simulink model "linearizzazione_pendolo_inv"  (R2020b)
settings: Solver=VariableStepAuto  StartTime=0.0  StopTime=20.0  RelTol=1e-3
values from neighbouring files (symbols this model uses):
  A = [0 1; -k/(m*L*L)+g/L*cos(x_bar(1)) -a/(m*L*L)]    [pendolo_inverso.m]
  B = [0 ; 0]    [pendolo_inverso.m]
  C = [1 0]    [pendolo_inverso.m]
  D = 0    [pendolo_inverso.m]
  du = u-u_bar    (= 0)    [pendolo_inverso.m]
  dx0 = x0-x_bar    [pendolo_inverso.m]
  x_bar = [0.713; 0]    [pendolo_inverso.m]
settings Model: Creator=Lenovo  LastModifiedBy=Lenovo

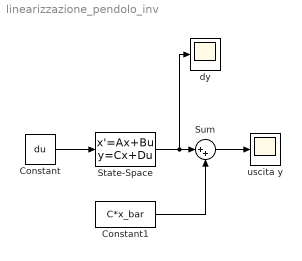
== system linearizzazione_pendolo_inv ==
  Constant : Constant  Value=du
  Constant1 : Constant  Value=C*x_bar
  State-Space : StateSpace  A=A  B=B  C=C  D=D  InitialCondition=dx0
  Sum : Sum  Inputs=|++
  dy : Scope
  uscita y : Scope
  wires:
  Constant/1 -> State-Space/1
  State-Space/1 -> dy/1, Sum/1
  Constant1/1 -> Sum/2
  Sum/1 -> uscita y/1
